simulink model "rtwdemo_lct_gain"  (Simulink 7.6)
settings: Solver=FixedStepDiscrete  StartTime=0.0  StopTime=10.0  FixedStep=1  RelTol=1e-3
libraries: rtwdemowidgets x2
Description:
  | Return Arguments
settings Model: Creator=The MathWorks Inc.  ExtModeAutoUpdateStatusClock=off
settings MATStruct: SampleTime=1  Offset=0  Priority=[20.0]
settings DataIOCC: SaveOutput=off  SaveTime=off  SignalLoggingName=logsOut
settings OptimizationCC: InlineParams=on  InlineInvariantSignals=on  EfficientFloat2IntCast=on  EfficientMapNaN2IntZero=off
settings DebuggingCC: SolverPrmCheckMsg=none  StrictBusMsg=ErrorOnBusTreatedAsVector
settings HardwareCC: ProdIntDivRoundTo=Zero  ProdEndianess=LittleEndian  ProdHWDeviceType=Generic->32-bit Embedded Processor  TargetHWDeviceType=Generic->32-bit Embedded Processor
settings RTWCC: GenerateReport=on  RTWVerbose=off  ProcessScript=grt_make_rtw_hook  LaunchReport=on
settings GRTTargetCC: TargetFcnLib=ansi_tfl_tmw.mat

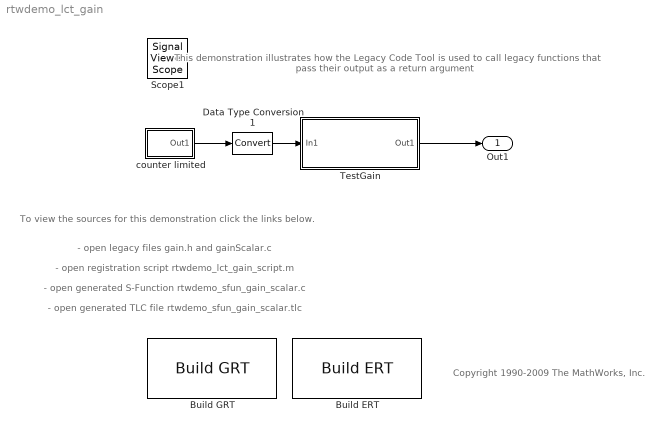
== system rtwdemo_lct_gain ==
  note: Copyright 1990-2009 The MathWorks, Inc.
  note: This demonstration illustrates how the Legacy Code Tool is used to
      | call legacy functions that pass their output as a return argument
  note: - open legacy files gain.h and gainScalar.c
  note: To view the sources for this demonstration
      | click the links below.
  note: - open registration script rtwdemo_lct_gain_script.m
  note: - open generated S-Function rtwdemo_sfun_gain_scalar.c
  note: - open generated TLC file rtwdemo_sfun_gain_scalar.tlc
  Build ERT : rtwdemowidgets/Build ERT  SystemSampleTime=-1  attrib_overrides={}
  Build GRT : rtwdemowidgets/Build GRT  SystemSampleTime=-1  attrib_overrides={}
  Data Type Conversion1 : DataTypeConversion  RndMeth=Zero
  TestGain : Subsystem
  counter limited : Subsystem  mask(CounterLimited){th=2^16-1}
      mask prompts: th "Threshold:"
  Out1 : Outport
  Scope1 : SignalViewerScope  IOType=viewer  RefreshTime=0.035000
      settings: YMin=0  YMax=120
  wires:
  TestGain/1(Out1) -> Out1/1
  counter limited/1(Out1) -> Data Type Conversion1/1
  Data Type Conversion1/1 -> TestGain/1(In1)

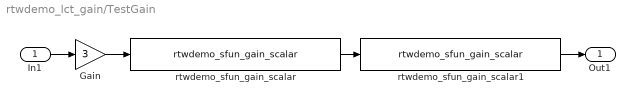
== system rtwdemo_lct_gain/TestGain ==
  In1 : Inport
  Gain : Gain  Gain=3  OutDataTypeStr=Inherit: Inherit via back propagation
  rtwdemo_sfun_gain_scalar : S-Function  FunctionName=rtwdemo_sfun_gain_scalar  Parameters=SParameter1  EnableBusSupport=off  mask(Legacy Function){SFunctionSpec=single y1 = gainScalar(single u1, single p1), SParameter1=single(2), ShowSpec=on}
      mask prompts: SParameter1 "P1:"; ShowSpec "Display function specification"
      mask help:
      | This block allows you to call the legacy functions specified by the following Legacy Code Tool definition:
      | def.SFunctionName = 'rtwdemo_sfun_gain_scalar';
      | def.OutputFcnSpec = 'single y1 = gainScalar(single u1, single p1)';
      | def.HeaderFiles = {'gain.h'};
      | def.SourceFiles = {'gainScalar.c'};
      | def.IncPaths = {'sldemo_lct_src'};
      | def.SrcPaths = {'sldemo_lct_src'};
      mask Help: <p>This block was generated automatically by the Legacy Code Tool. For detailed help on this tool, call<a href="matlab:legacy_code('help')"> legacy_code('help')</a>.</p>
      mask CallbackString:
      | ||if strcmp(get_param(gcbh, 'ShowSpec'), 'on')
      |   set_param(gcbh, 'MaskDisplay', sprintf('fprintf(''%s'');', get_param(gcbh, 'SFunctionSpec')));
      | else
      |   set_param(gcbh, 'MaskDisplay', sprintf('fprintf(''%s'');', get_param(gcbh, 'FunctionName')));
      | end
      mask Display: fprintf('single y1 = gainScalar(single u1, single p1)');
  rtwdemo_sfun_gain_scalar1 : S-Function  FunctionName=rtwdemo_sfun_gain_scalar  Parameters=SParameter1  EnableBusSupport=off  mask(Legacy Function){SFunctionSpec=single y1 = gainScalar(single u1, single p1), SParameter1=single(2), ShowSpec=on}
      mask prompts: SParameter1 "P1:"; ShowSpec "Display function specification"
      mask help:
      | This block allows you to call the legacy functions specified by the following Legacy Code Tool definition:
      | def.SFunctionName = 'rtwdemo_sfun_gain_scalar';
      | def.OutputFcnSpec = 'single y1 = gainScalar(single u1, single p1)';
      | def.HeaderFiles = {'gain.h'};
      | def.SourceFiles = {'gainScalar.c'};
      | def.IncPaths = {'sldemo_lct_src'};
      | def.SrcPaths = {'sldemo_lct_src'};
      mask Help: <p>This block was generated automatically by the Legacy Code Tool. For detailed help on this tool, call<a href="matlab:legacy_code('help')"> legacy_code('help')</a>.</p>
      mask CallbackString:
      | ||if strcmp(get_param(gcbh, 'ShowSpec'), 'on')
      |   set_param(gcbh, 'MaskDisplay', sprintf('fprintf(''%s'');', get_param(gcbh, 'SFunctionSpec')));
      | else
      |   set_param(gcbh, 'MaskDisplay', sprintf('fprintf(''%s'');', get_param(gcbh, 'FunctionName')));
      | end
      mask Display: fprintf('single y1 = gainScalar(single u1, single p1)');
  Out1 : Outport
  wires:
  Gain/1 -> rtwdemo_sfun_gain_scalar/1
  In1/1 -> Gain/1
  rtwdemo_sfun_gain_scalar/1 -> rtwdemo_sfun_gain_scalar1/1
  rtwdemo_sfun_gain_scalar1/1 -> Out1/1

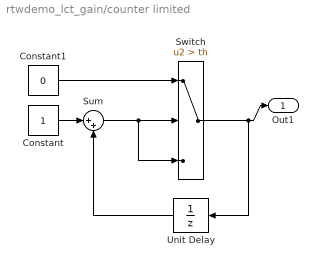
== system rtwdemo_lct_gain/counter limited ==
  Constant : Constant
  Constant1 : Constant  Value=0
  Sum : Sum  Inputs=|++
  Switch : Switch  Criteria=u2 > Threshold  Threshold=th  ZeroCross=off
  Unit Delay : UnitDelay  X0=-1  SampleTime=-1
  Out1 : Outport
  wires:
  Constant/1 -> Sum/1
  Sum/1 -> Switch/2, Switch/3
  Unit Delay/1 -> Sum/2
  Constant1/1 -> Switch/1
  Switch/1 -> Unit Delay/1, Out1/1
